simulink model "power_harmonicfilter"  (Simulink 6.0)
settings: Solver=FixedStepDiscrete  SolverMode=SingleTasking  StartTime=0.0  StopTime=0.1  FixedStep=Ts  MaxStep=1/512/60  RelTol=1e-4
PreLoadFcn:
  | Ts=1/512/60;
undefined symbols (not defined in the file or in its folder): D1, Delta
libraries: powerlib x17, powerlib_extras x3
settings Model: Creator=hyp01  LastModifiedBy=batserve  ExtModeAutoUpdateStatusClock=off
settings DataIOCC: LimitDataPoints=off  SignalLoggingName=sigsOut
settings DebuggingCC: CheckExecutionContextPreStartOutputMsg=on  CheckExecutionContextRuntimeOutputMsg=on  SolverPrmCheckMsg=none  UnconnectedLineMsg=none
settings HardwareCC: TargetUnknown=on

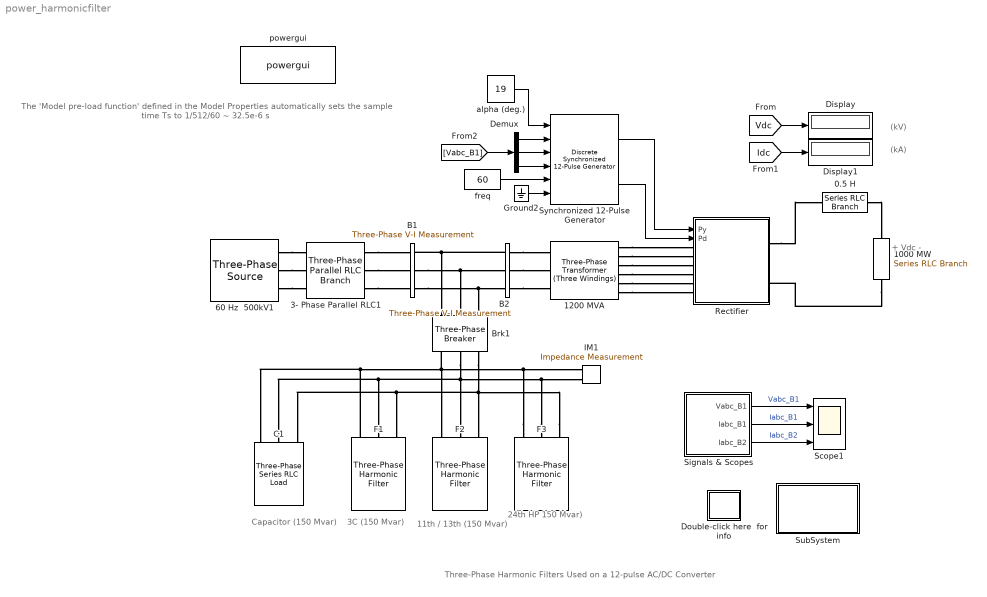
== system power_harmonicfilter ==
  note: 11th / 13th
      | (150 Mvar)
  note: 24th HP
      | 150 Mvar)
  note: The 'Model  pre-load function' defined in the
      | Model Properties automatically sets the sample time
      | Ts to 1/512/60 ~ 32.5e-6 s
  note: +
      |
      |
      | Vdc
      |
      |
      | -
  note: 3C
      | (150 Mvar)
  note: Capacitor
      | (150 Mvar)
  note: (kV)
  note: (kA)
  note: Three-Phase Harmonic Filters Used on a 12-pulse AC/DC Converter
  " 60 Hz  500kV1" : powerlib/Electrical Sources/Three-Phase Source  Voltage=500e3  PhaseAngle=0  Frequency=60  InternalConnection=Yg  SpecifyImpedance=off  Resistance=0  Inductance=98.03e-3  ShortCircuitLevel=0  BaseVoltage=0  XRratio=0
  "0.5 H " : powerlib/Elements/Series RLC Branch  PhysicalDomain=powersysdomain  SubClassName=unknown  LeftPortType=p1  RightPortType=p1  LConnTagsString=__new0  RConnTagsString=__new0  Resistance=1  Inductance=0.5  Capacitance=inf  Measurements=None
  1000 MW : powerlib/Elements/Series RLC Branch  Orientation=down  PhysicalDomain=powersysdomain  SubClassName=unknown  LeftPortType=p1  RightPortType=p1  LConnTagsString=__new0  RConnTagsString=__new0  Resistance=500e3^2/1000e6  Inductance=0  Capacitance=inf  Measurements=Branch voltage and current
  1200 MVA : powerlib/Elements/Three-Phase Transformer (Three Windings)  NominalPower=[ 1200e6 , 60 ]  Winding1Connection=Yg  Winding1="[ 500e3*0.9 0.0025  0 ]"  Winding2Connection=Y  Winding2=[ 200e3 0.0025 0.24]  Winding3Connection=Delta (D1)  Winding3=[ 200e3 0.0025 0.24 ]  SetSaturation=off  Rm=500  Lm=500  Saturation=[0 0; 1 1.2; 2 1.1]  Hysteresis=off  DataFile='hysteresis'  SetInitialFlux=off  InitialFluxes=[0.8 -0.8 0.7]  Measurements=All measurements (V I Fluxes)  TransfoNumber=0
      settings: AttributesFormatString=\n
  3- Phase Parallel RLC1 : powerlib/Elements/Three-Phase Parallel RLC Branch  PhysicalDomain=powersysdomain  SubClassName=unknown  LeftPortType=p1  RightPortType=p1  LConnTagsString=A|B|C  RConnTagsString=A|B|C  Resistance=26.07  Inductance=48.86e-3  Capacitance=0  Measurements=None
  B1 : powerlib/Measurements/Three-Phase V-I Measurement  VoltageMeasurement=phase-to-ground  SetLabelV=on  LabelV=Vabc_B1  Vpu=off  Vbase=500e3  CurrentMeasurement=yes  SetLabelI=on  LabelI=Iabc_B1  Ipu=off  Pbase=100e6  OutputType=Magnitude  PhasorSimulation=off  PSBequivalent=0
  "B2 " : powerlib/Measurements/Three-Phase V-I Measurement  VoltageMeasurement=phase-to-ground  SetLabelV=on  LabelV=Vabc_B2  Vpu=off  Vbase=500e3  CurrentMeasurement=yes  SetLabelI=on  LabelI=Iabc_B2  Ipu=off  Pbase=100e6  OutputType=Magnitude  PhasorSimulation=off  PSBequivalent=0
  Brk1 : powerlib/Elements/Three-Phase Breaker  Orientation=down  InitialState=closed  SwitchA=off  SwitchB=off  SwitchC=off  SwitchTimes="[4/60  10/60]"  External=off  BreakerResistance=1e-4  SnubberResistance=1e6  SnubberCapacitance=inf  Measurements=None
      settings: AttributesFormatString=\n
  C1 : powerlib/Elements/Three-Phase Series RLC Load  Orientation=down  PhysicalDomain=powersysdomain  SubClassName=unknown  LeftPortType=p1  RightPortType=p1  LConnTagsString=A|B|C  Configuration=Y (grounded)  NominalVoltage=500e3  NominalFrequency=60  ActivePower=0  InductivePower=0  CapacitivePower=150e6  Measurements=None
  Demux : Demux  Outputs=3
  Display : Display
      settings: Format=bank  SampleTime=Ts*20
  Display1 : Display
      settings: Format=bank  SampleTime=Ts*20
  Double-click here  for info : Subsystem
      mask Display: disp('?')
  "F1 " : powerlib/Elements/Three-Phase Harmonic Filter  Orientation=down  PhysicalDomain=powersysdomain  SubClassName=unknown  LeftPortType=p1  RightPortType=p1  LConnTagsString=A|B|C  FilterType=C-type High-pass  FilterConnection=Y (grounded)  ParNom=[500e3 60]  Qc=150e6  Fr=[3*60]  Frd=[11*60 13*60]  Q=2  Measurements=None
      settings: AttributesFormatString=\n
  F2 : powerlib/Elements/Three-Phase Harmonic Filter  Orientation=down  PhysicalDomain=powersysdomain  SubClassName=unknown  LeftPortType=p1  RightPortType=p1  LConnTagsString=A|B|C  FilterType=Double-tuned  FilterConnection=Y (grounded)  ParNom=[500e3 60]  Qc=150e6  Fr=[3*60]  Frd=[11*60 13*60]  Q=20  Measurements=None
      settings: AttributesFormatString=\n
  F3 : powerlib/Elements/Three-Phase Harmonic Filter  Orientation=down  PhysicalDomain=powersysdomain  SubClassName=unknown  LeftPortType=p1  RightPortType=p1  LConnTagsString=A|B|C  FilterType=High-pass  FilterConnection=Y (grounded)  ParNom=[500e3 60]  Qc=150e6  Fr=[24*60]  Frd=[11*60 13*60]  Q=7  Measurements=None
      settings: AttributesFormatString=\n
  Ground2 : Ground
  IM1 : powerlib/Measurements/Impedance Measurement  PhysicalDomain=powersysdomain  SubClassName=unknown  LeftPortType=p1  RightPortType=p1  LConnTagsString=+|-  RConnTagsString=__newr0  Factor=0.5
      settings: AttributesFormatString=\n
  Rectifier : Subsystem
      mask Display: plot(0,0,100,100,[30 70 50 30 ], [40 40 60 40], [50 50], [25 40], [50 50], [ 60 75], [30 70], [60 60], [50 40 30], [60 70 70]);
  Scope1 : Scope  NumInputPorts=3
      settings: YMin=-600000~-2500~-2500  YMax=600000~2500~2500  SaveName=Scope1
  "Signals & Scopes " : Subsystem
  SubSystem : Subsystem
      settings: OpenFcn=openfig('filters_impedance.fig');
      mask Display: disp('Show\nfilters impedance\nvs\nfrequency')
  Synchronized 12-Pulse Generator : powerlib_extras/Discrete  Control Blocks/Discrete Synchronized 12-Pulse Generator  pwidth=40  Double_Pulse=on  Ts=Ts
  alpha (deg.) : Constant  Value=19
  freq : Constant  Value=60
  powergui : powerlib/powergui  Priority=2  Frange=[50:2:3000]  Ylog=off  Xlog=off  save=on  variable=ZData5  structure=Scope1  ZoomFFT=on  StartTime=0.06  cycles=2  DisplayStyle=1  fundamental=60  FreqAxis=off  MaxFrequency=4000  frequencyindice=1  frequencyindicesteady=1  RmsSteady=1  display=off  Ts=Ts  methode=off  frequency=60  echomessages=on
  wires:
  [Vdc] -> Display/1
  [Idc] -> Display1/1
  freq/1 -> Synchronized 12-Pulse Generator/5
  Ground2/1 -> Synchronized 12-Pulse Generator/6
  Demux/1 -> Synchronized 12-Pulse Generator/2
  Demux/2 -> Synchronized 12-Pulse Generator/3
  Demux/3 -> Synchronized 12-Pulse Generator/4
  [Vabc_B1] -> Demux/1
  Synchronized 12-Pulse Generator/1 -> Rectifier/1(Py)
  Synchronized 12-Pulse Generator/2 -> Rectifier/2(Pd)
  alpha (deg.)/1 -> Synchronized 12-Pulse Generator/1
  "Signals & Scopes "/1(Vabc_B1) -> Scope1/1  "Vabc_B1"
  "Signals & Scopes "/2(Iabc_B1) -> Scope1/2  "Iabc_B1"
  "Signals & Scopes "/3(Iabc_B2) -> Scope1/3  "Iabc_B2"
  connections:
  Rectifier/RConn1 -- "0.5 H "/LConn1
  "0.5 H "/RConn1 -- 1000 MW/LConn1
  1000 MW/RConn1 -- Rectifier/RConn2
  1200 MVA/RConn1 -- Rectifier/LConn1
  1200 MVA/RConn2 -- Rectifier/LConn2
  1200 MVA/RConn3 -- Rectifier/LConn3
  1200 MVA/RConn4 -- Rectifier/LConn4
  1200 MVA/RConn5 -- Rectifier/LConn5
  1200 MVA/RConn6 -- Rectifier/LConn6
  "B2 "/LConn1 -- B1/RConn1 -- Brk1/LConn1
  B1/RConn2 -- "B2 "/LConn2 -- Brk1/LConn2
  B1/RConn3 -- "B2 "/LConn3 -- Brk1/LConn3
  F3/LConn1 -- C1/LConn1 -- "F1 "/LConn1 -- Brk1/RConn1 -- F2/LConn1 -- IM1/LConn1
  F3/LConn2 -- C1/LConn2 -- "F1 "/LConn2 -- Brk1/RConn2 -- F2/LConn2 -- IM1/LConn2
  "B2 "/RConn2 -- 1200 MVA/LConn2
  "B2 "/RConn1 -- 1200 MVA/LConn1
  "B2 "/RConn3 -- 1200 MVA/LConn3
  " 60 Hz  500kV1"/RConn2 -- 3- Phase Parallel RLC1/LConn2
  " 60 Hz  500kV1"/RConn3 -- 3- Phase Parallel RLC1/LConn3
  " 60 Hz  500kV1"/RConn1 -- 3- Phase Parallel RLC1/LConn1
  3- Phase Parallel RLC1/RConn1 -- B1/LConn1
  3- Phase Parallel RLC1/RConn2 -- B1/LConn2
  3- Phase Parallel RLC1/RConn3 -- B1/LConn3
  F3/LConn3 -- C1/LConn3 -- "F1 "/LConn3 -- Brk1/RConn3 -- F2/LConn3

== system power_harmonicfilter/Double-click here  for info ==
  note: Run a first simulation with an alpha firing angle of 19 degrees. You should get a DC voltage level of 500 kV.
      | Now, look inside Scope1. Compare the currents flowing into Bus B1 (Iabc_B1, axis 2) with those flowing into Bus B2 (Iabc_B2, axis 3).
      | You can see that the harmonic filters almost eliminate the harmonics generated by the converter. If you use the FFT tool of the powergui,
      | you will find that the harmonic filters reduce the THD of the current injected in the system from 9% to 0.7%.
      | You can also perform other simulations with various values of alpha. Notice the impact on the DC level and on the generated harmonics.
  note: Pierre Giroux (Hydro-Quebec)
  note: Frequency response
  note: CIRCUIT DESCRIPTION
  note: Three-Phase Harmonic Filters
  note: The HVDC rectifier is built up from two 6-pulse thyristor bridges connected in series. The converter is connected to the system
      | with a 1200-MVA Three-Phase  transformer (three windings). A 1000-MW resistive load is connected to the DC side through
      | a 0.5 H smoothing reactor.
      | The filters set is made of the following four components of the powerlib/Elements library:
      | - one capacitor banks (C1) of 150 Mvar modeled by a "Three-Phase Series RLC Load",
      | - three filters modeled using the "Three-Phase Harmonic Filter"
      |             - one C-type high-pass filter tuned to the 3rd (F1) of 150 Mvar
      |             - one double-tuned filter 11/13 th (F2) of 150 Mvar
      |             - one high-pass filter tuned to the 24th (F3) of 150 Mvar
      | The total Mvar rating of the filters set is then 600 Mvar.
      | A three-phase circuit breaker (Brk1) is used to connect the filters set on the AC bus.
      |
      | The converter is open-loop controlled using the "Synchronized 12-Pulse Generator"
      | of the Extras/Discrete Control library with a constant conduction angle alpha of 19 degrees.
  note: DEMONSTRATION
  note: Time-domain simulation
  note: You will now plot the impedance vs frequency of the harmonic filters:
      | 1) Disconnect the filters from the AC bus. To do so, double-click on the breaker Brk1, select 'open' for initial status of breakers
      | and click on the OK button.
      | 2) Open the powergui and select "Impedance vs Frequency Measurement".
      | 3) Click on the Display/Save button. SimPowerSystems will compute and display the filters frequency response.
      | 4) Double-click on the block "Show filters impedance vs frequency". A second figure, showing the pre-computed filters
      | frequency response will be displayed. The impedance data of the two figures should be identical.
      | 5) If you zoom the figure (using the "Tool" menu), you should find an impedance of 417 ohms capacitive (-90deg.) at 60 Hz.
      | This value confirms that the total reactive power of the filters at 60 Hz is: Qc =V^2/Xc = 500e3^2/417 = 600 Mvar.
  note: In HVDC installations, AC harmonic shunt filters are used to:
      | 1)  reduce harmonic voltages and currents in the power system,
      | 2)  supply the reactive power consumed by the converter.
      | To illustrate these concepts, a 1000-MW (500 kV, 2kA) HVDC rectifier is simulated.

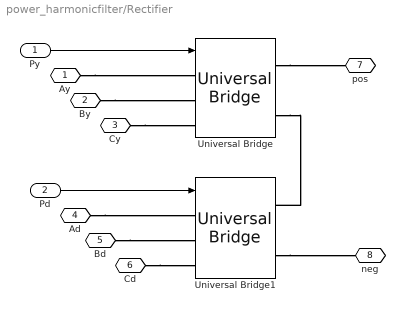
== system power_harmonicfilter/Rectifier ==
  Py : Inport  Port=1  LatchInput=off
  Pd : Inport  Port=2  LatchInput=off
  Universal Bridge : powerlib/Power Electronics/Universal Bridge  Arms=3  SnubberResistance=2000  SnubberCapacitance=0.1e-6  Device=Thyristors  Ron=1e-3  Lon=0  ForwardVoltages="[  0.8  0.8  ]"  ForwardVoltage=0  GTOparameters=[ 10e-6 , 20e-6 ]  IGBTparameters=[ 1e-6 , 2e-6 ]  Measurements=None
  Universal Bridge1 : powerlib/Power Electronics/Universal Bridge  Arms=3  SnubberResistance=2000  SnubberCapacitance=0.1e-6  Device=Thyristors  Ron=1e-3  Lon=0  ForwardVoltages="[  0.8  0.8  ]"  ForwardVoltage=0  GTOparameters=[ 10e-6 , 20e-6 ]  IGBTparameters=[ 1e-6 , 2e-6 ]  Measurements=None
  Ay : PMIOPort  Port=1  Side=Left
  By : PMIOPort  Port=2  Side=Left
  Cy : PMIOPort  Port=3  Side=Left
  Ad : PMIOPort  Port=4  Side=Left
  Bd : PMIOPort  Port=5  Side=Left
  Cd : PMIOPort  Port=6  Side=Left
  pos : PMIOPort  Orientation=left  Port=7  Side=Right
  neg : PMIOPort  Orientation=left  Port=8  Side=Right
  wires:
  Py/1 -> Universal Bridge/1
  Pd/1 -> Universal Bridge1/1
  connections:
  Ay/RConn1 -- Universal Bridge/LConn1
  Universal Bridge/RConn1 -- pos/RConn1
  Cy/RConn1 -- Universal Bridge/LConn3
  Ad/RConn1 -- Universal Bridge1/LConn1
  Bd/RConn1 -- Universal Bridge1/LConn2
  Cd/RConn1 -- Universal Bridge1/LConn3
  Universal Bridge1/RConn2 -- neg/RConn1
  By/RConn1 -- Universal Bridge/LConn2
  Universal Bridge/RConn2 -- Universal Bridge1/RConn1

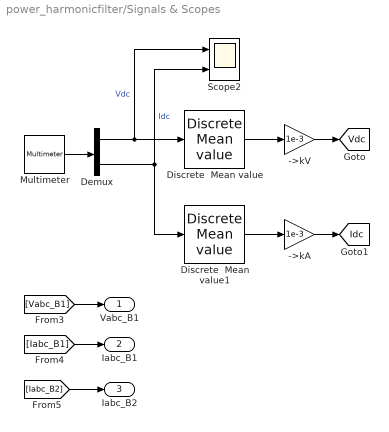
== system power_harmonicfilter/Signals & Scopes  ==
  ->kA : Gain  Gain=1e-3  SaturateOnIntegerOverflow=on
  ->kV : Gain  Gain=1e-3  SaturateOnIntegerOverflow=on
  Demux : Demux  Outputs=[1 1]
  Discrete  Mean value : powerlib_extras/Discrete Measurements/Discrete  Mean value  Freq=60  Vinit=0  Ts=Ts
  Discrete  Mean value1 : powerlib_extras/Discrete Measurements/Discrete  Mean value  Freq=60  Vinit=0  Ts=Ts
  Multimeter : powerlib/Measurements/Multimeter  PhasorSimulation=off  OutputType=Magnitude  sel=[1 11]  L=23  Gain=[1 1]  yselected={'Ub: 1000 MW','Ib: 1000 MW'};  PSBOutputType=1  PSBequivalent=0  AxesSetting=[0,0.1,-100,100]  Display=0  SavedBlockNames=-11
  Scope2 : Scope  NumInputPorts=2
      settings: YMin=-25000~-100  YMax=525000~2100
  Vabc_B1 : Outport
  Iabc_B1 : Outport  Port=2
  Iabc_B2 : Outport  Port=3
  tag scope: Idc=global, Vdc=global
  wires:
  Multimeter/1 -> Demux/1
  ->kV/1 -> [Vdc]
  Discrete  Mean value/1 -> ->kV/1
  Discrete  Mean value1/1 -> ->kA/1
  ->kA/1 -> [Idc]
  Demux/1 -> Discrete  Mean value/1, Scope2/1  "Vdc"
  Demux/2 -> Discrete  Mean value1/1, Scope2/2  "Idc"
  [Vabc_B1] -> Vabc_B1/1
  [Iabc_B1] -> Iabc_B1/1
  [Iabc_B2] -> Iabc_B2/1

== system power_harmonicfilter/SubSystem ==
